simulink library "INT_EGRVlv_VDMon"  (R2016b)
settings: Solver=VariableStepAuto  StartTime=0.0  StopTime=10.0  RelTol=1e-3
settings Model: Creator=zhulinfeng  LastModifiedBy=zhulinfeng

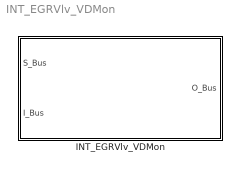
== system INT_EGRVlv_VDMon ==
  INT_EGRVlv_VDMon : Subsystem

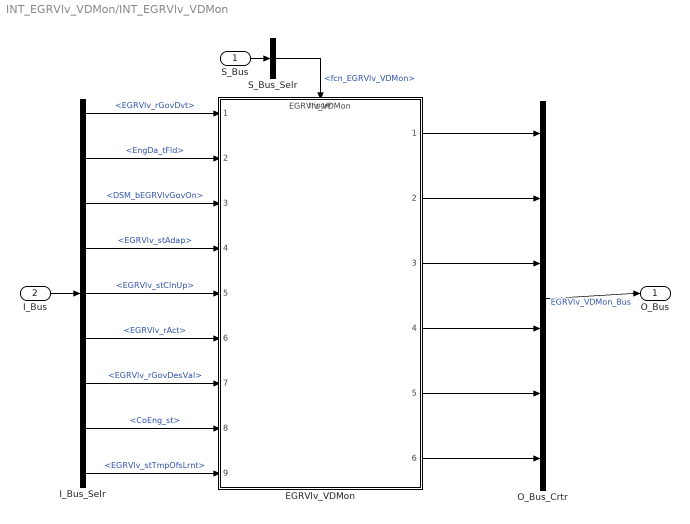
== system INT_EGRVlv_VDMon/INT_EGRVlv_VDMon ==
  S_Bus : Inport
  I_Bus : Inport  Port=2
  EGRVlv_VDMon : ModelReference  ModelNameDialog=EGRVlv_VDMon  SimulationMode=Normal  ModelReferenceVersion=1.16  TriggerPortName=function  TriggerPortTriggerType=function-call  TriggerPortStatesWhenEnabling=held
  I_Bus_Selr : BusSelector  OutputSignals=EGRVlv_rGovDvt,EngDa_tFld,DSM_bEGRVlvGovOn,EGRVlv_stAdap,EGRVlv_stClnUp,EGRVlv_rAct,EGRVlv_rGovDesVal,CoEng_st,EGRVlv_stTmpOfsLrnt
  O_Bus_Crtr : BusCreator  Inputs=6
  S_Bus_Selr : BusSelector  OutputSignals=fcn_EGRVlv_VDMon
  O_Bus : Outport
  wires:
  S_Bus_Selr/1 -> EGRVlv_VDMon/Trigger  "<fcn_EGRVlv_VDMon>"
  S_Bus/1 -> S_Bus_Selr/1
  I_Bus/1 -> I_Bus_Selr/1
  I_Bus_Selr/1 -> EGRVlv_VDMon/1  "<EGRVlv_rGovDvt>"
  I_Bus_Selr/2 -> EGRVlv_VDMon/2  "<EngDa_tFld>"
  I_Bus_Selr/3 -> EGRVlv_VDMon/3  "<DSM_bEGRVlvGovOn>"
  I_Bus_Selr/4 -> EGRVlv_VDMon/4  "<EGRVlv_stAdap>"
  I_Bus_Selr/5 -> EGRVlv_VDMon/5  "<EGRVlv_stClnUp>"
  I_Bus_Selr/6 -> EGRVlv_VDMon/6  "<EGRVlv_rAct>"
  I_Bus_Selr/7 -> EGRVlv_VDMon/7  "<EGRVlv_rGovDesVal>"
  I_Bus_Selr/8 -> EGRVlv_VDMon/8  "<CoEng_st>"
  I_Bus_Selr/9 -> EGRVlv_VDMon/9  "<EGRVlv_stTmpOfsLrnt>"
  O_Bus_Crtr/1 -> O_Bus/1  "EGRVlv_VDMon_Bus"
  EGRVlv_VDMon/1 -> O_Bus_Crtr/1
  EGRVlv_VDMon/2 -> O_Bus_Crtr/2
  EGRVlv_VDMon/3 -> O_Bus_Crtr/3
  EGRVlv_VDMon/4 -> O_Bus_Crtr/4
  EGRVlv_VDMon/5 -> O_Bus_Crtr/5
  EGRVlv_VDMon/6 -> O_Bus_Crtr/6
